simulink model "verify_Ground_Source_Heat_Exchanger_mdl"  (R2016b)
settings: Solver=ode45  StartTime=0  StopTime=2*3600  MaxStep=600  RelTol=1e-3  EnableMultiTasking=on
InitFcn:
  | load('DE_TRY2010_13_averageYear')
libraries: carnot x3
settings Model: Creator=drhf  LastModifiedBy=User
settings DataIOCC: SaveFormat=Array  SignalLoggingSaveFormat=ModelDataLogs
settings OptimizationCC: ExpressionDepthLimit=2147483647  LifeSpan=inf
settings DebuggingCC: UnderspecifiedInitializationDetection=Classic  MergeDetectMultiDrivingBlocksExec=none  SolverPrmCheckMsg=warning  FcnCallInpInsideContextMsg=warning  StateNameClashWarn=warning  SFUnexpectedBacktrackingDiag=warning  SFNoUnconditionalDefaultTransitionDiag=warning  SFExecutionAtInitializationDiag=none
settings HardwareCC: ProdBitPerPointer=32  ProdBitPerSizeT=32  ProdBitPerPtrDiffT=32  ProdLargestAtomicFloat=None  ProdIntDivRoundTo=Undefined  ProdEndianess=Unspecified  ProdWordSize=32  ProdHWDeviceType=32-bit Generic
settings ModelReferenceCC: PropagateSignalLabelsOutOfModel=off
settings GRTTargetCC: TargetLangStandard=C89/C90 (ANSI)  GeneratePreprocessorConditionals=Disable all  CombineOutputUpdateFcns=off  GRTInterface=on
settings ConfigComp: CovMetricSettings=dw  CovHtmlReporting=on  CovSaveCumulativeToWorkspaceVar=on  CovSaveSingleToWorkspaceVar=on  CovExternalEMLEnable=off

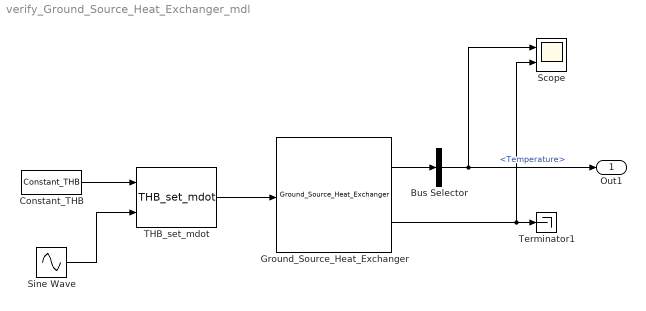
== system verify_Ground_Source_Heat_Exchanger_mdl ==
  Bus Selector : BusSelector  OutputSignals=Temperature
  Constant_THB : carnot/Source/Simple/Constant_THB  t=40  mdot=50/3600  p=1e5  mID=No Pressure Drop  fluid=Water  mix=0  mix2=0  mix3=0  dia=0.02  hgt=0
  Ground_Source_Heat_Exchanger : carnot/Source/Heat_Pump/Ground_Source_Heat_Exchanger  Jahresmitteltemp_C=12  TGrad=0.025  lambdaErde=2.0  cpErde=800  rhoErde=2500  lambdaFill=1.0  cpFill=1000  rhoFill=2000  Sondelaenge=100  B=10  Sondendurchmesser=0.032  Bohrdurchmesser=0.18  sondenfall=1 probe  np=1  DimAxi=10  DimRad=10  Gitterfaktor=2.5
  Scope : Scope  NumInputPorts=2
  Sine Wave : Sin  Amplitude=500/3600  Bias=400/3600  Frequency=2*pi/3600  SampleTime=0
  THB_set_mdot : carnot/Source/Simple/THB_set_mdot
  Terminator1 : Terminator
  Out1 : Outport
  wires:
  Ground_Source_Heat_Exchanger/1 -> Bus Selector/1
  Constant_THB/1 -> THB_set_mdot/1
  Sine Wave/1 -> THB_set_mdot/2
  THB_set_mdot/1 -> Ground_Source_Heat_Exchanger/1
  Bus Selector/1 -> Scope/1, Out1/1  "<Temperature>"
  Ground_Source_Heat_Exchanger/2 -> Scope/2, Terminator1/1
